simulink model "sl_quadrotor"  (Simulink 8.4)
settings: Solver=ode45  StartTime=0.0  StopTime=3  MaxStep=0.1  RelTol=1e-3
InitFcn:
  | % load parameters of the default quadrotor
  | disp('Quadrotor parameters loaded by InitFcn')
  | quad_param
  | ctrl_param
  | des_traj
values from neighbouring files (symbols this model uses):
  enable_plot = true    [run_model.m]
undefined symbols (not defined in the file or in its folder): ctrl, quad
settings Model: Creator=corkep  LastModifiedBy=zichao

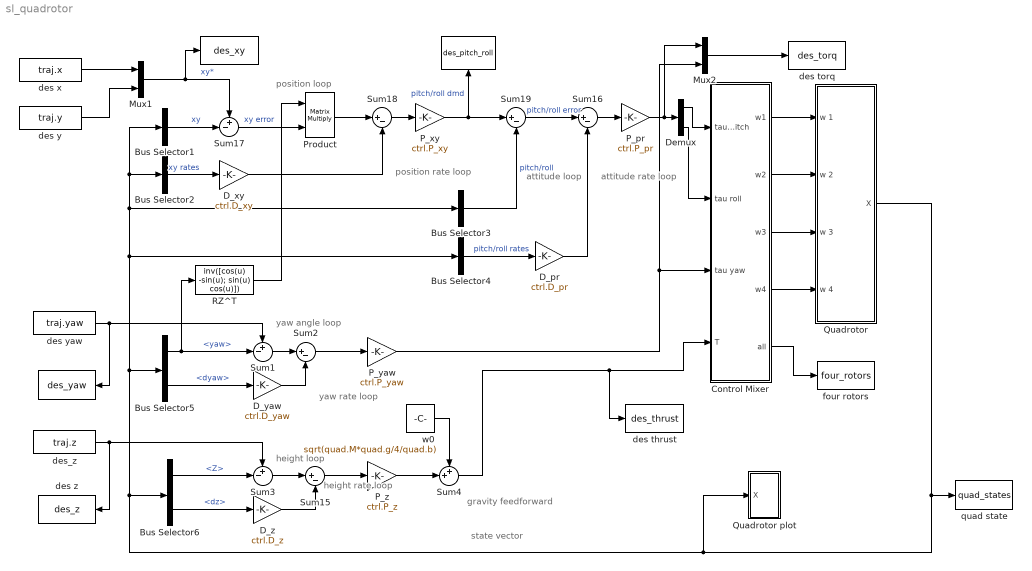
== system sl_quadrotor ==
  note: state vector
  note: gravity feedforward
  note: attitude rate
      | loop
  note: attitude
      | loop
  note: position rate
      | loop
  note: position
      | loop
  note: yaw rate
      | loop
  note: yaw angle
      | loop
  note: height rate
      | loop
  note: height
      | loop
  " " : ToWorkspace  VariableName=des_xy  SaveFormat=Timeseries  SampleTime=-1
  "  " : ToWorkspace  VariableName=des_yaw  SaveFormat=Timeseries  SampleTime=-1
  "   " : ToWorkspace  VariableName=des_pitch_roll  SaveFormat=Timeseries  SampleTime=-1
  " des z" : ToWorkspace  VariableName=des_z  SaveFormat=Timeseries  SampleTime=-1
  Bus Selector1 : BusSelector  OutputSignals=X,Y  OutputAsBus=on
  Bus Selector2 : BusSelector  OutputSignals=dx,dy  OutputAsBus=on
  Bus Selector3 : BusSelector  OutputSignals=pitch,roll  OutputAsBus=on
  Bus Selector4 : BusSelector  OutputSignals=dpitch,droll  OutputAsBus=on
  Bus Selector5 : BusSelector  OutputSignals=yaw,dyaw
  Bus Selector6 : BusSelector  OutputSignals=Z,dz
  Control Mixer : Subsystem
      mask help: Quadrotor control mixer
      mask Help:
      | Determine rotor speeds based on desired torques and thrust.
      | 
      | <b>Inputs::</b>
      | 
      | tau pitch (1x1)  desired pitching torque [Nm]
      | tau roll (1x1)   desired rolling torque [Nm]
      | tau yaw (1x1)    desired yawing torque [Nm]
      | T (1x1)          desired thrust [N]
      | 
      | <b>Outputs::</b>
      | 
      | w1 (1x1) angular velocity of rotor 1 [rad]
      | w2 (1x1) angular velocity of rotor 2 [rad]
      | w3 (1x1) angular velocity of rotor 3 [rad]
      | w4 (1x1) angular velocity of rotor 4 [rad]
      | 
      | <b>Notes::</b>
      | 
      | - Assumes the rotor labelling convention of RVC Fig 4.16.
      | - The quadrotor is underactuated and has only 4 inputs.
  D_pr : Gain  Gain=ctrl.D_pr
  D_xy : Gain  Gain=ctrl.D_xy
  D_yaw : Gain  Gain=ctrl.D_yaw
  D_z : Gain  Gain=ctrl.D_z
  Demux : Demux  Outputs=2
  Mux1 : Mux  Inputs=2
  Mux2 : Mux  Inputs=2
  P_pr : Gain  Gain=ctrl.P_pr
  P_xy : Gain  Gain=ctrl.P_xy
  P_yaw : Gain  Gain=ctrl.P_yaw
  P_z : Gain  Gain=ctrl.P_z
  Product : Product  Multiplication=Matrix(*)  RndMeth=Zero
  Quadrotor : Subsystem  mask{quad=quad}
      mask prompts: quad "Quadrotor params"
      mask help: Quadrotor dynamics
      mask Help:
      | Integrate spatial velocity to update pose represented as a homogeneous
      | transformation.
      | 
      | <b>Parameters::</b>
      | 
      | q (struct)  A structure containing quadrotor dynamics
      | 
      | The elements of q are:
      | 
      |  J         Flyer rotational inertia matrix (3x3)
      |  h         Height of rotors above CoG (1x1)
      |  d         Length of flyer arms (1x1)
      |  nb        Number of blades per rotor (1x1)
      |  r         Rotor radius (1x1)
      |  c         Blade chord (1x1)
      |  e         Flapping hinge offset (1x1)
      |  Mb        Rotor blade mass (1x1)
      |  Mc        Estimated hub clamp mass (1x1)
      |  ec        Blade root clamp displacement (1x1)
      |  Ib        Rotor blade rotational inertia (1x1)
      |  Ic        Estimated root clamp inertia (1x1)
      |  mb        Static blade moment (1x1)
      |  Ir        Total rotor inertia (1x1)
      |  Ct        Non-dim. thrust coefficient (1x1)
      |  Cq        Non-dim. torque coefficient (1x1)
      |  sigma     Rotor solidity ratio (1x1)
      |  thetat    Blade tip angle (1x1)
      |  theta0    Blade root angle (1x1)
      |  theta1    Blade twist angle (1x1)
      |  theta75   3/4 blade angle (1x1)
      |  thetai    Blade ideal root approximation (1x1)
      |  a         Lift slope gradient (1x1)
      |  A         Rotor disc area (1x1)
      |  gamma     Lock number (1x1)
      | 
      | 
      | <b>Inputs::</b>
      | 
      | w1 (1x1) angular velocity of rotor 1 [rad]
      | w2 (1x1) angular velocity of rotor 2 [rad]
      | w3 (1x1) angular velocity of rotor 3 [rad]
      | w4 (1x1) angular velocity of rotor 4 [rad]
      | 
      | <b>Outputs::</b>
      | 
      | X (1x12) state vector (x, y, z, thr, thp, thy, xd, yd, zd, thrd, thpd, thyd)
      | 
      | (x,y,z) is the position in the world frame [m]
      | (thr, thp, thy) the roll/pitch/yaw orientation in the world frame [rad]
      | (xd,yd,zd) is the velocity in the body frame [m]
      | (thrd,thpd,thyd) is the roll/pitch/yaw rates in the body frame [rad/s]
      | 
      | <b>Notes::</b>
      | 
      | - See also mdl_quadrotor which defines parameters for the ANU X4 flyer.
  Quadrotor plot : Subsystem
  RZ^T : MATLABFcn  MATLABFcn=inv([cos(u) -sin(u); sin(u) cos(u)])  OutputDimensions=[2 2]  Output1D=off
  Sum1 : Sum  Inputs=+-|
  Sum{2,15..16,18..19} (5 alike) : Sum  Inputs=|+-
  Sum17 : Sum  Inputs=+-|
  Sum3 : Sum  Inputs=+-|
  Sum4 : Sum  Inputs=++|
  des thrust : ToWorkspace  VariableName=des_thrust  SaveFormat=Timeseries  SampleTime=-1
  des torq : ToWorkspace  VariableName=des_torq  SaveFormat=Timeseries  SampleTime=-1
  des x : FromWorkspace  VariableName=traj.x  SampleTime=0
  des y : FromWorkspace  VariableName=traj.y  SampleTime=0
  des yaw : FromWorkspace  VariableName=traj.yaw  SampleTime=0
  des_z : FromWorkspace  VariableName=traj.z  SampleTime=0
  four rotors : ToWorkspace  VariableName=four_rotors  SaveFormat=Timeseries  SampleTime=-1
  quad state : ToWorkspace  VariableName=quad_states  SaveFormat=Timeseries  SampleTime=-1
  w0 : Constant  Value=sqrt(quad.M*quad.g/4/quad.b)  SampleTime=0
  wires:
  Control Mixer/1(w1) -> Quadrotor/1(w 1)
  Control Mixer/4(w4) -> Quadrotor/4(w 4)
  w0/1 -> Sum4/1
  Sum15/1 -> P_z/1
  P_z/1 -> Sum4/2
  Quadrotor/1(X) -> quad state/1, Quadrotor plot/1(X), Bus Selector6/1, Bus Selector4/1, Bus Selector3/1, Bus Selector1/1, Bus Selector2/1, Bus Selector5/1
  Bus Selector1/1 -> Sum17/2  "xy"
  Mux1/1 -> " "/1, Sum17/1  "xy*"
  Bus Selector2/1 -> D_xy/1  "xy rates"
  D_xy/1 -> Sum18/2
  P_xy/1 -> Sum19/1, "   "/1  "pitch/roll dmd"
  Bus Selector3/1 -> Sum19/2  "pitch/roll"
  Bus Selector4/1 -> D_pr/1  "pitch/roll rates"
  Sum19/1 -> Sum16/1  "pitch/roll error"
  Sum16/1 -> P_pr/1
  P_pr/1 -> Mux2/1, Demux/1
  P_yaw/1 -> Mux2/2, Control Mixer/3(tau yaw)
  Bus Selector5/1 -> RZ^T/1, Sum1/2  "<yaw>"
  Sum2/1 -> P_yaw/1
  Bus Selector6/1 -> Sum3/2  "<Z>"
  des_z/1 -> " des z"/1, Sum3/1
  Bus Selector5/2 -> D_yaw/1  "<dyaw>"
  Sum3/1 -> Sum15/1
  Bus Selector6/2 -> D_z/1  "<dz>"
  D_z/1 -> Sum15/2
  D_pr/1 -> Sum16/2
  Demux/2 -> Control Mixer/2(tau roll)
  D_yaw/1 -> Sum2/2
  Sum4/1 -> des thrust/1, Control Mixer/4(T)
  Sum1/1 -> Sum2/1
  Sum18/1 -> P_xy/1
  des yaw/1 -> "  "/1, Sum1/1
  Product/1 -> Sum18/1
  Sum17/1 -> Product/2  "xy error"
  RZ^T/1 -> Product/1
  Demux/1 -> Control Mixer/1(tau pitch)
  Control Mixer/3(w3) -> Quadrotor/3(w 3)
  Control Mixer/2(w2) -> Quadrotor/2(w 2)
  Control Mixer/5(all) -> four rotors/1
  Mux2/1 -> des torq/1
  des x/1 -> Mux1/1
  des y/1 -> Mux1/2

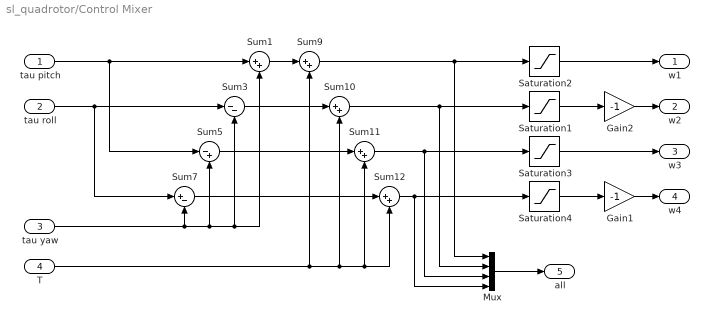
== system sl_quadrotor/Control Mixer ==
  tau pitch : Inport
  tau roll : Inport  Port=2
  tau yaw : Inport  Port=3
  T : Inport  Port=4
  Gain1 : Gain  Gain=-1
  Gain2 : Gain  Gain=-1
  Mux : Mux
  Saturation{1..4} (4 alike) : Saturate  UpperLimit=1000  LowerLimit=700
  Sum{1,9..12} (5 alike) : Sum  Inputs=|++  SaturateOnIntegerOverflow=on  InputSameDT=on  OutDataTypeStr=Inherit: Same as first input
  Sum3 : Sum  Inputs=|--  SaturateOnIntegerOverflow=on  InputSameDT=on  OutDataTypeStr=Inherit: Same as first input
  Sum5 : Sum  Inputs=|-+  SaturateOnIntegerOverflow=on  InputSameDT=on  OutDataTypeStr=Inherit: Same as first input
  Sum7 : Sum  Inputs=|+-  SaturateOnIntegerOverflow=on  InputSameDT=on  OutDataTypeStr=Inherit: Same as first input
  w1 : Outport
  w2 : Outport  Port=2
  w3 : Outport  Port=3
  w4 : Outport  Port=4
  all : Outport  Port=5
  wires:
  tau yaw/1 -> Sum7/2, Sum5/2, Sum3/2, Sum1/2
  Saturation2/1 -> w1/1
  Saturation1/1 -> Gain2/1
  Saturation3/1 -> w3/1
  Saturation4/1 -> Gain1/1
  tau pitch/1 -> Sum1/1, Sum5/1
  Sum1/1 -> Sum9/1
  Sum3/1 -> Sum10/1
  Sum5/1 -> Sum11/1
  Sum7/1 -> Sum12/1
  Sum9/1 -> Saturation2/1, Mux/1
  Sum10/1 -> Saturation1/1, Mux/2
  Sum11/1 -> Saturation3/1, Mux/3
  Sum12/1 -> Saturation4/1, Mux/4
  T/1 -> Sum12/2, Sum11/2, Sum10/2, Sum9/2
  tau roll/1 -> Sum3/1, Sum7/1
  Mux/1 -> all/1
  Gain2/1 -> w2/1
  Gain1/1 -> w4/1

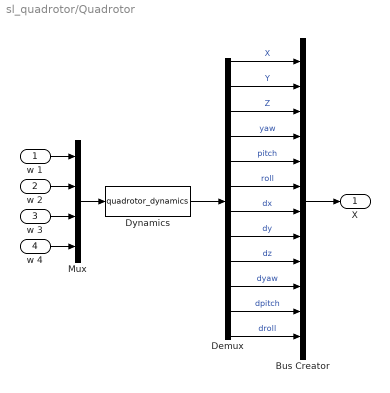
== system sl_quadrotor/Quadrotor ==
  w 1 : Inport
  w 2 : Inport  Port=2
  w 3 : Inport  Port=3
  w 4 : Inport  Port=4
  Bus Creator : BusCreator  Inputs='X','Y','Z','yaw','pitch','roll','dx','dy','dz','dyaw','dpitch','droll'
  Demux : Demux  Outputs=12
  Dynamics : S-Function  FunctionName=quadrotor_dynamics  Parameters=quad  EnableBusSupport=off
  Mux : Mux
  X : Outport
  wires:
  Mux/1 -> Dynamics/1
  Demux/1 -> Bus Creator/1  "X"
  Demux/3 -> Bus Creator/3  "Z"
  Demux/4 -> Bus Creator/4  "yaw"
  Demux/5 -> Bus Creator/5  "pitch"
  w 1/1 -> Mux/1
  w 2/1 -> Mux/2
  w 3/1 -> Mux/3
  w 4/1 -> Mux/4
  Demux/7 -> Bus Creator/7  "dx"
  Demux/9 -> Bus Creator/9  "dz"
  Demux/2 -> Bus Creator/2  "Y"
  Demux/6 -> Bus Creator/6  "roll"
  Demux/8 -> Bus Creator/8  "dy"
  Bus Creator/1 -> X/1
  Dynamics/1 -> Demux/1
  Demux/10 -> Bus Creator/10  "dyaw"
  Demux/11 -> Bus Creator/11  "dpitch"
  Demux/12 -> Bus Creator/12  "droll"

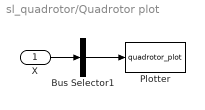
== system sl_quadrotor/Quadrotor plot ==
  X : Inport
  Bus Selector1 : BusSelector  OutputSignals=X,Y,Z,yaw,pitch,roll  OutputAsBus=on
  Plotter : S-Function  FunctionName=quadrotor_plot  Parameters=[2, 10], 1, enable_plot  EnableBusSupport=off
  wires:
  X/1 -> Bus Selector1/1
  Bus Selector1/1 -> Plotter/1
